simulink model "FullEKF_2010a"  (Simulink 6.6)
settings: Solver=FixedStepDiscrete  StartTime=0.0  StopTime=300  FixedStep=0.01  RelTol=1e-3
values from neighbouring files (symbols this model uses):
  initP = diag([1e-3 1e-3 1e-3 1e-6 1e-6 1e-6 1 1 1 5e-6 5e-6 5e-6 1e-8 1e-8 1e-8])    [FullEKF_init.m.m]
undefined symbols (not defined in the file or in its folder): DiscIntNeverNeededParam, gcbh, hwbcalib_subsystem
libraries: simulink x6, dspmtrx3 x4, dspinverses x1
(part 4 of 7)

== system FullEKF_2010a/Trajectory  Generator/Signals Conversions dtgen/Subsystem1 ==
  note: Equation for Transforming Geodetic Coordinate
      | to Rectangular (ECEF) coordinates:
      | (NIMA TR8350.2 Third Edition, 3 January 2000)
      |
      | Equation 4-14:
      | x_{ECEF} = (N + h)cos(\lambda)cos(\Lambda)
      | y_{ECEF} = (N + h)cos(\lambda)sin(\Lambda)
      | z_{ECEF} = ((b/a)^2N + h)sin(\lambda)
      |
      | Equation 4-15:
      | N = a / (1-e^2sin^2(\lambda))^{1/2}
      |
      | Where:
      | (\lambda, \Lambda, h) = geodetic coordinates (in meters & rad)
      | b/a = earth axis ratio
      | a = earth semi-major axis (in m)
      | e = earth first eccentricity
  geoToECEFLibInLon : Inport  OutDataType=fixdt(1,16,0)  OutScaling=[]
  geoToECEFLibInLat : Inport  Port=2  OutDataType=fixdt(1,16,0)  OutScaling=[]
  geoToECEFLibInAlt : Inport  Port=3  OutDataType=fixdt(1,16,0)  OutScaling=[]
  Math Function : Math  Operator=reciprocal  OutDataType=fixdt(1,16,0)  OutScaling=[]  SaturateOnIntegerOverflow=on
  Sqrt : Math  Operator=sqrt  OutDataType=fixdt(1,16,0)  OutScaling=[]  SaturateOnIntegerOverflow=on
  Trigonometric Function : Trigonometry  Operator=cos
  Trigonometric Function1 : Trigonometry  Operator=cos
  Trigonometric Function2 : Trigonometry
  Trigonometric Function3 : Trigonometry
  axisRatio : Gain  Tag=MBDLibrary v2007b.1  Gain=.996647189335^2  ParameterDataType=fixdt(1,16,0)  ParameterScaling=[]  OutDataType=fixdt(1,16,0)  OutScaling=[]  RndMeth=Zero  mask(Gain (MBDLibrary)){gain_mbdlib=.996647189335^2}
      mask prompts: gain_mbdlib "Gain"
      mask help: Multiplies the input by the gain.
      settings: OpenFcn=|
      | if exist('mbdlib_dialog')
      |    mbdlib_dialog(gcb,'open')
      | else
      |    open_system(gcb, 'mask')
      | end
      mask Help: The GAIN block multiplies the input by the gain value.  This block may accept any data types other than boolean.  The user must take care to not use a non-integer gain for int32/uint32 inputs.
      mask Display: disp([get_param(gcb, 'Gain') 'x'])
  bias : Bias  Tag=MBDLibrary v2007b.1  Bias=1  mask(Bias (MBDLibrary)){Bias_mbdlib=1}
      mask prompts: Bias_mbdlib "Bias"
      mask help: Add bias to input.
      settings: OpenFcn=|
      | if exist('mbdlib_dialog')
      |    mbdlib_dialog(gcb,'open')
      | else
      |    open_system(gcb, 'mask')
      | end
      settings: CloseFcn=|
      | if exist('mbdlib_bias')
      |    mbdlib_bias(gcb)
      | end
      mask Help: The BIAS block outputs the summation of an input with a specified constant.
      mask Display: disp(['x+1'])
  eqPlane : Product  Tag=MBDLibrary v2007b.1  OutDataType=fixdt(1,16,0)  OutScaling=[]  RndMeth=Zero  InputSameDT=on  mask(Product (MBDLibrary)){Inputs_mbdlib=2}
      mask prompts: Inputs_mbdlib "Number of Inputs"
      mask help: Multiplies inputs.
      settings: OpenFcn=|
      | if exist('mbdlib_dialog')
      |    mbdlib_dialog(gcb,'open')
      | else
      |    open_system(gcb, 'mask')
      | end
      mask Help: The PRODUCT block is used to multiply inputs.
  firstEccentricitySquared : Gain  Tag=MBDLibrary v2007b.1  Gain=-6.69437999014e-3  ParameterDataType=fixdt(1,16,0)  ParameterScaling=[]  OutDataType=fixdt(1,16,0)  OutScaling=[]  RndMeth=Zero  mask(Gain (MBDLibrary)){gain_mbdlib=-6.69437999014e-3}
      mask prompts: gain_mbdlib "Gain"
      mask help: Multiplies the input by the gain.
      settings: OpenFcn=|
      | if exist('mbdlib_dialog')
      |    mbdlib_dialog(gcb,'open')
      | else
      |    open_system(gcb, 'mask')
      | end
      mask Help: The GAIN block multiplies the input by the gain value.  This block may accept any data types other than boolean.  The user must take care to not use a non-integer gain for int32/uint32 inputs.
      mask Display: disp([get_param(gcb, 'Gain') 'x'])
  gain : Gain  Tag=MBDLibrary v2007b.1  Gain=6378137.0  ParameterDataType=fixdt(1,16,0)  ParameterScaling=[]  OutDataType=fixdt(1,16,0)  OutScaling=[]  RndMeth=Zero  mask(Gain (MBDLibrary)){gain_mbdlib=6378137.0}
      mask prompts: gain_mbdlib "Gain"
      mask help: Multiplies the input by the gain.
      settings: OpenFcn=|
      | if exist('mbdlib_dialog')
      |    mbdlib_dialog(gcb,'open')
      | else
      |    open_system(gcb, 'mask')
      | end
      mask Help: The GAIN block multiplies the input by the gain value.  This block may accept any data types other than boolean.  The user must take care to not use a non-integer gain for int32/uint32 inputs.
      mask Display: disp([get_param(gcb, 'Gain') 'x'])
  radius : Sum  Tag=MBDLibrary v2007b.1  OutDataType=fixdt(1,16,0)  OutScaling=[]  RndMeth=Zero  InputSameDT=on  mask(Sum (MBDLibrary)){inputs_mbdlib=++}
      mask prompts: inputs_mbdlib "List of signs"
      mask help: Adds values together.
      settings: OpenFcn=|
      | if exist('mbdlib_dialog')
      |    mbdlib_dialog(gcb,'open')
      | else
      |    open_system(gcb, 'mask')
      | end
      mask Help:
      | The SUM block is used to add or subtract  inputs.
      | The inputs may be specified as:
      |   (a) + or - for each port (i.e. ++-+)
      |   (b) An integer to indicate the number of ports to add
      | Note that the number of ports input to this block must be between 1 and 25.
      | When only 1 inport is selected, the block computes the summation of vector input elements and outputs a scalar.
  radius1 : Sum  Tag=MBDLibrary v2007b.1  OutDataType=fixdt(1,16,0)  OutScaling=[]  RndMeth=Zero  InputSameDT=on  mask(Sum (MBDLibrary)){inputs_mbdlib=++}
      mask prompts: inputs_mbdlib "List of signs"
      mask help: Adds values together.
      settings: OpenFcn=|
      | if exist('mbdlib_dialog')
      |    mbdlib_dialog(gcb,'open')
      | else
      |    open_system(gcb, 'mask')
      | end
      mask Help:
      | The SUM block is used to add or subtract  inputs.
      | The inputs may be specified as:
      |   (a) + or - for each port (i.e. ++-+)
      |   (b) An integer to indicate the number of ports to add
      | Note that the number of ports input to this block must be between 1 and 25.
      | When only 1 inport is selected, the block computes the summation of vector input elements and outputs a scalar.
  square : Subsystem  Tag=MBDLibrary v2007b.1
      settings: OpenFcn=|
      | if exist('mbdlib_dialog')
      |    mbdlib_dialog(gcb,'open')
      | else
      |    open_system(gcb, 'mask')
      | end
      mask Type: Square (MBDLibrary)
      mask Description: Squares the input.
      mask Help: The SQAURE block outputs the square of the input value.
      mask Display: disp('x^2', 'texmode', 'on')
  xECEF : Product  Tag=MBDLibrary v2007b.1  OutDataType=fixdt(1,16,0)  OutScaling=[]  RndMeth=Zero  InputSameDT=on  mask(Product (MBDLibrary)){Inputs_mbdlib=2}
      mask prompts: Inputs_mbdlib "Number of Inputs"
      mask help: Multiplies inputs.
      settings: OpenFcn=|
      | if exist('mbdlib_dialog')
      |    mbdlib_dialog(gcb,'open')
      | else
      |    open_system(gcb, 'mask')
      | end
      mask Help: The PRODUCT block is used to multiply inputs.
  yECEF : Product  Tag=MBDLibrary v2007b.1  OutDataType=fixdt(1,16,0)  OutScaling=[]  RndMeth=Zero  InputSameDT=on  mask(Product (MBDLibrary)){Inputs_mbdlib=2}
      mask prompts: Inputs_mbdlib "Number of Inputs"
      mask help: Multiplies inputs.
      settings: OpenFcn=|
      | if exist('mbdlib_dialog')
      |    mbdlib_dialog(gcb,'open')
      | else
      |    open_system(gcb, 'mask')
      | end
      mask Help: The PRODUCT block is used to multiply inputs.
  zECEF : Product  Tag=MBDLibrary v2007b.1  OutDataType=fixdt(1,16,0)  OutScaling=[]  RndMeth=Zero  InputSameDT=on  mask(Product (MBDLibrary)){Inputs_mbdlib=2}
      mask prompts: Inputs_mbdlib "Number of Inputs"
      mask help: Multiplies inputs.
      settings: OpenFcn=|
      | if exist('mbdlib_dialog')
      |    mbdlib_dialog(gcb,'open')
      | else
      |    open_system(gcb, 'mask')
      | end
      mask Help: The PRODUCT block is used to multiply inputs.
  geoToECEFLibOutX : Outport  OutDataType=fixdt(1,16,0)  OutScaling=[]
  geoToECEFLibOutY : Outport  Port=2  OutDataType=fixdt(1,16,0)  OutScaling=[]
  geoToECEFLibOutZ : Outport  Port=3  OutDataType=fixdt(1,16,0)  OutScaling=[]
  wires:
  Trigonometric Function3/1 -> zECEF/2, square/1(squareLibIn)
  zECEF/1 -> geoToECEFLibOutZ/1
  yECEF/1 -> geoToECEFLibOutY/1
  xECEF/1 -> geoToECEFLibOutX/1
  radius1/1 -> zECEF/1
  eqPlane/1 -> yECEF/2, xECEF/1
  Trigonometric Function2/1 -> yECEF/1
  geoToECEFLibInLon/1 -> Trigonometric Function1/1, Trigonometric Function2/1
  axisRatio/1 -> radius1/2
  geoToECEFLibInAlt/1 -> radius1/1, radius/2
  gain/1 -> axisRatio/1, radius/1
  Trigonometric Function/1 -> eqPlane/1
  Trigonometric Function1/1 -> xECEF/2
  radius/1 -> eqPlane/2
  bias/1 -> Sqrt/1
  firstEccentricitySquared/1 -> bias/1
  square/1(squareLibOut) -> firstEccentricitySquared/1
  geoToECEFLibInLat/1 -> Trigonometric Function/1, Trigonometric Function3/1
  Sqrt/1 -> Math Function/1
  Math Function/1 -> gain/1

== system FullEKF_2010a/EKF/MeasureVector/GPS/Subsystem1 ==
  note: Equation for Transforming Geodetic Coordinate
      | to Rectangular (ECEF) coordinates:
      | (NIMA TR8350.2 Third Edition, 3 January 2000)
      |
      | Equation 4-14:
      | x_{ECEF} = (N + h)cos(\lambda)cos(\Lambda)
      | y_{ECEF} = (N + h)cos(\lambda)sin(\Lambda)
      | z_{ECEF} = ((b/a)^2N + h)sin(\lambda)
      |
      | Equation 4-15:
      | N = a / (1-e^2sin^2(\lambda))^{1/2}
      |
      | Where:
      | (\lambda, \Lambda, h) = geodetic coordinates (in meters & rad)
      | b/a = earth axis ratio
      | a = earth semi-major axis (in m)
      | e = earth first eccentricity
  geoToECEFLibInLon : Inport  OutDataType=fixdt(1,16,0)  OutScaling=[]
  geoToECEFLibInLat : Inport  Port=2  OutDataType=fixdt(1,16,0)  OutScaling=[]
  geoToECEFLibInAlt : Inport  Port=3  OutDataType=fixdt(1,16,0)  OutScaling=[]
  Math Function : Math  Operator=reciprocal  OutDataType=fixdt(1,16,0)  OutScaling=[]  SaturateOnIntegerOverflow=on
  Sqrt : Math  Operator=sqrt  OutDataType=fixdt(1,16,0)  OutScaling=[]  SaturateOnIntegerOverflow=on
  Trigonometric Function : Trigonometry  Operator=cos
  Trigonometric Function1 : Trigonometry  Operator=cos
  Trigonometric Function2 : Trigonometry
  Trigonometric Function3 : Trigonometry
  axisRatio : Gain  Tag=MBDLibrary v2007b.1  Gain=.996647189335^2  ParameterDataType=fixdt(1,16,0)  ParameterScaling=[]  OutDataType=fixdt(1,16,0)  OutScaling=[]  RndMeth=Zero  mask(Gain (MBDLibrary)){gain_mbdlib=.996647189335^2}
      mask prompts: gain_mbdlib "Gain"
      mask help: Multiplies the input by the gain.
      settings: OpenFcn=|
      | if exist('mbdlib_dialog')
      |    mbdlib_dialog(gcb,'open')
      | else
      |    open_system(gcb, 'mask')
      | end
      mask Help: The GAIN block multiplies the input by the gain value.  This block may accept any data types other than boolean.  The user must take care to not use a non-integer gain for int32/uint32 inputs.
      mask Display: disp([get_param(gcb, 'Gain') 'x'])
  bias : Bias  Tag=MBDLibrary v2007b.1  Bias=1  mask(Bias (MBDLibrary)){Bias_mbdlib=1}
      mask prompts: Bias_mbdlib "Bias"
      mask help: Add bias to input.
      settings: OpenFcn=|
      | if exist('mbdlib_dialog')
      |    mbdlib_dialog(gcb,'open')
      | else
      |    open_system(gcb, 'mask')
      | end
      settings: CloseFcn=|
      | if exist('mbdlib_bias')
      |    mbdlib_bias(gcb)
      | end
      mask Help: The BIAS block outputs the summation of an input with a specified constant.
      mask Display: disp(['x+1'])
  eqPlane : Product  Tag=MBDLibrary v2007b.1  OutDataType=fixdt(1,16,0)  OutScaling=[]  RndMeth=Zero  InputSameDT=on  mask(Product (MBDLibrary)){Inputs_mbdlib=2}
      mask prompts: Inputs_mbdlib "Number of Inputs"
      mask help: Multiplies inputs.
      settings: OpenFcn=|
      | if exist('mbdlib_dialog')
      |    mbdlib_dialog(gcb,'open')
      | else
      |    open_system(gcb, 'mask')
      | end
      mask Help: The PRODUCT block is used to multiply inputs.
  firstEccentricitySquared : Gain  Tag=MBDLibrary v2007b.1  Gain=-6.69437999014e-3  ParameterDataType=fixdt(1,16,0)  ParameterScaling=[]  OutDataType=fixdt(1,16,0)  OutScaling=[]  RndMeth=Zero  mask(Gain (MBDLibrary)){gain_mbdlib=-6.69437999014e-3}
      mask prompts: gain_mbdlib "Gain"
      mask help: Multiplies the input by the gain.
      settings: OpenFcn=|
      | if exist('mbdlib_dialog')
      |    mbdlib_dialog(gcb,'open')
      | else
      |    open_system(gcb, 'mask')
      | end
      mask Help: The GAIN block multiplies the input by the gain value.  This block may accept any data types other than boolean.  The user must take care to not use a non-integer gain for int32/uint32 inputs.
      mask Display: disp([get_param(gcb, 'Gain') 'x'])
  gain : Gain  Tag=MBDLibrary v2007b.1  Gain=6378137.0  ParameterDataType=fixdt(1,16,0)  ParameterScaling=[]  OutDataType=fixdt(1,16,0)  OutScaling=[]  RndMeth=Zero  mask(Gain (MBDLibrary)){gain_mbdlib=6378137.0}
      mask prompts: gain_mbdlib "Gain"
      mask help: Multiplies the input by the gain.
      settings: OpenFcn=|
      | if exist('mbdlib_dialog')
      |    mbdlib_dialog(gcb,'open')
      | else
      |    open_system(gcb, 'mask')
      | end
      mask Help: The GAIN block multiplies the input by the gain value.  This block may accept any data types other than boolean.  The user must take care to not use a non-integer gain for int32/uint32 inputs.
      mask Display: disp([get_param(gcb, 'Gain') 'x'])
  radius : Sum  Tag=MBDLibrary v2007b.1  OutDataType=fixdt(1,16,0)  OutScaling=[]  RndMeth=Zero  InputSameDT=on  mask(Sum (MBDLibrary)){inputs_mbdlib=++}
      mask prompts: inputs_mbdlib "List of signs"
      mask help: Adds values together.
      settings: OpenFcn=|
      | if exist('mbdlib_dialog')
      |    mbdlib_dialog(gcb,'open')
      | else
      |    open_system(gcb, 'mask')
      | end
      mask Help:
      | The SUM block is used to add or subtract  inputs.
      | The inputs may be specified as:
      |   (a) + or - for each port (i.e. ++-+)
      |   (b) An integer to indicate the number of ports to add
      | Note that the number of ports input to this block must be between 1 and 25.
      | When only 1 inport is selected, the block computes the summation of vector input elements and outputs a scalar.
  radius1 : Sum  Tag=MBDLibrary v2007b.1  OutDataType=fixdt(1,16,0)  OutScaling=[]  RndMeth=Zero  InputSameDT=on  mask(Sum (MBDLibrary)){inputs_mbdlib=++}
      mask prompts: inputs_mbdlib "List of signs"
      mask help: Adds values together.
      settings: OpenFcn=|
      | if exist('mbdlib_dialog')
      |    mbdlib_dialog(gcb,'open')
      | else
      |    open_system(gcb, 'mask')
      | end
      mask Help:
      | The SUM block is used to add or subtract  inputs.
      | The inputs may be specified as:
      |   (a) + or - for each port (i.e. ++-+)
      |   (b) An integer to indicate the number of ports to add
      | Note that the number of ports input to this block must be between 1 and 25.
      | When only 1 inport is selected, the block computes the summation of vector input elements and outputs a scalar.
  square : Subsystem  Tag=MBDLibrary v2007b.1
      settings: OpenFcn=|
      | if exist('mbdlib_dialog')
      |    mbdlib_dialog(gcb,'open')
      | else
      |    open_system(gcb, 'mask')
      | end
      mask Type: Square (MBDLibrary)
      mask Description: Squares the input.
      mask Help: The SQAURE block outputs the square of the input value.
      mask Display: disp('x^2', 'texmode', 'on')
  xECEF : Product  Tag=MBDLibrary v2007b.1  OutDataType=fixdt(1,16,0)  OutScaling=[]  RndMeth=Zero  InputSameDT=on  mask(Product (MBDLibrary)){Inputs_mbdlib=2}
      mask prompts: Inputs_mbdlib "Number of Inputs"
      mask help: Multiplies inputs.
      settings: OpenFcn=|
      | if exist('mbdlib_dialog')
      |    mbdlib_dialog(gcb,'open')
      | else
      |    open_system(gcb, 'mask')
      | end
      mask Help: The PRODUCT block is used to multiply inputs.
  yECEF : Product  Tag=MBDLibrary v2007b.1  OutDataType=fixdt(1,16,0)  OutScaling=[]  RndMeth=Zero  InputSameDT=on  mask(Product (MBDLibrary)){Inputs_mbdlib=2}
      mask prompts: Inputs_mbdlib "Number of Inputs"
      mask help: Multiplies inputs.
      settings: OpenFcn=|
      | if exist('mbdlib_dialog')
      |    mbdlib_dialog(gcb,'open')
      | else
      |    open_system(gcb, 'mask')
      | end
      mask Help: The PRODUCT block is used to multiply inputs.
  zECEF : Product  Tag=MBDLibrary v2007b.1  OutDataType=fixdt(1,16,0)  OutScaling=[]  RndMeth=Zero  InputSameDT=on  mask(Product (MBDLibrary)){Inputs_mbdlib=2}
      mask prompts: Inputs_mbdlib "Number of Inputs"
      mask help: Multiplies inputs.
      settings: OpenFcn=|
      | if exist('mbdlib_dialog')
      |    mbdlib_dialog(gcb,'open')
      | else
      |    open_system(gcb, 'mask')
      | end
      mask Help: The PRODUCT block is used to multiply inputs.
  geoToECEFLibOutX : Outport  OutDataType=fixdt(1,16,0)  OutScaling=[]
  geoToECEFLibOutY : Outport  Port=2  OutDataType=fixdt(1,16,0)  OutScaling=[]
  geoToECEFLibOutZ : Outport  Port=3  OutDataType=fixdt(1,16,0)  OutScaling=[]
  wires:
  Trigonometric Function3/1 -> zECEF/2, square/1(squareLibIn)
  zECEF/1 -> geoToECEFLibOutZ/1
  yECEF/1 -> geoToECEFLibOutY/1
  xECEF/1 -> geoToECEFLibOutX/1
  radius1/1 -> zECEF/1
  eqPlane/1 -> yECEF/2, xECEF/1
  Trigonometric Function2/1 -> yECEF/1
  geoToECEFLibInLon/1 -> Trigonometric Function1/1, Trigonometric Function2/1
  axisRatio/1 -> radius1/2
  geoToECEFLibInAlt/1 -> radius1/1, radius/2
  gain/1 -> axisRatio/1, radius/1
  Trigonometric Function/1 -> eqPlane/1
  Trigonometric Function1/1 -> xECEF/2
  radius/1 -> eqPlane/2
  bias/1 -> Sqrt/1
  firstEccentricitySquared/1 -> bias/1
  square/1(squareLibOut) -> firstEccentricitySquared/1
  geoToECEFLibInLat/1 -> Trigonometric Function/1, Trigonometric Function3/1
  Sqrt/1 -> Math Function/1
  Math Function/1 -> gain/1

== system FullEKF_2010a/EKF/MeasureVector/GPS/Subsystem2 ==
  note: Equation for Transforming Geodetic Coordinate
      | to Rectangular (ECEF) coordinates:
      | (NIMA TR8350.2 Third Edition, 3 January 2000)
      |
      | Equation 4-14:
      | x_{ECEF} = (N + h)cos(\lambda)cos(\Lambda)
      | y_{ECEF} = (N + h)cos(\lambda)sin(\Lambda)
      | z_{ECEF} = ((b/a)^2N + h)sin(\lambda)
      |
      | Equation 4-15:
      | N = a / (1-e^2sin^2(\lambda))^{1/2}
      |
      | Where:
      | (\lambda, \Lambda, h) = geodetic coordinates (in meters & rad)
      | b/a = earth axis ratio
      | a = earth semi-major axis (in m)
      | e = earth first eccentricity
  geoToECEFLibInLon : Inport  OutDataType=fixdt(1,16,0)  OutScaling=[]
  geoToECEFLibInLat : Inport  Port=2  OutDataType=fixdt(1,16,0)  OutScaling=[]
  geoToECEFLibInAlt : Inport  Port=3  OutDataType=fixdt(1,16,0)  OutScaling=[]
  Math Function : Math  Operator=reciprocal  OutDataType=fixdt(1,16,0)  OutScaling=[]  SaturateOnIntegerOverflow=on
  Sqrt : Math  Operator=sqrt  OutDataType=fixdt(1,16,0)  OutScaling=[]  SaturateOnIntegerOverflow=on
  Trigonometric Function : Trigonometry  Operator=cos
  Trigonometric Function1 : Trigonometry  Operator=cos
  Trigonometric Function2 : Trigonometry
  Trigonometric Function3 : Trigonometry
  axisRatio : Gain  Tag=MBDLibrary v2007b.1  Gain=.996647189335^2  ParameterDataType=fixdt(1,16,0)  ParameterScaling=[]  OutDataType=fixdt(1,16,0)  OutScaling=[]  RndMeth=Zero  mask(Gain (MBDLibrary)){gain_mbdlib=.996647189335^2}
      mask prompts: gain_mbdlib "Gain"
      mask help: Multiplies the input by the gain.
      settings: OpenFcn=|
      | if exist('mbdlib_dialog')
      |    mbdlib_dialog(gcb,'open')
      | else
      |    open_system(gcb, 'mask')
      | end
      mask Help: The GAIN block multiplies the input by the gain value.  This block may accept any data types other than boolean.  The user must take care to not use a non-integer gain for int32/uint32 inputs.
      mask Display: disp([get_param(gcb, 'Gain') 'x'])
  bias : Bias  Tag=MBDLibrary v2007b.1  Bias=1  mask(Bias (MBDLibrary)){Bias_mbdlib=1}
      mask prompts: Bias_mbdlib "Bias"
      mask help: Add bias to input.
      settings: OpenFcn=|
      | if exist('mbdlib_dialog')
      |    mbdlib_dialog(gcb,'open')
      | else
      |    open_system(gcb, 'mask')
      | end
      settings: CloseFcn=|
      | if exist('mbdlib_bias')
      |    mbdlib_bias(gcb)
      | end
      mask Help: The BIAS block outputs the summation of an input with a specified constant.
      mask Display: disp(['x+1'])
  eqPlane : Product  Tag=MBDLibrary v2007b.1  OutDataType=fixdt(1,16,0)  OutScaling=[]  RndMeth=Zero  InputSameDT=on  mask(Product (MBDLibrary)){Inputs_mbdlib=2}
      mask prompts: Inputs_mbdlib "Number of Inputs"
      mask help: Multiplies inputs.
      settings: OpenFcn=|
      | if exist('mbdlib_dialog')
      |    mbdlib_dialog(gcb,'open')
      | else
      |    open_system(gcb, 'mask')
      | end
      mask Help: The PRODUCT block is used to multiply inputs.
  firstEccentricitySquared : Gain  Tag=MBDLibrary v2007b.1  Gain=-6.69437999014e-3  ParameterDataType=fixdt(1,16,0)  ParameterScaling=[]  OutDataType=fixdt(1,16,0)  OutScaling=[]  RndMeth=Zero  mask(Gain (MBDLibrary)){gain_mbdlib=-6.69437999014e-3}
      mask prompts: gain_mbdlib "Gain"
      mask help: Multiplies the input by the gain.
      settings: OpenFcn=|
      | if exist('mbdlib_dialog')
      |    mbdlib_dialog(gcb,'open')
      | else
      |    open_system(gcb, 'mask')
      | end
      mask Help: The GAIN block multiplies the input by the gain value.  This block may accept any data types other than boolean.  The user must take care to not use a non-integer gain for int32/uint32 inputs.
      mask Display: disp([get_param(gcb, 'Gain') 'x'])
  gain : Gain  Tag=MBDLibrary v2007b.1  Gain=6378137.0  ParameterDataType=fixdt(1,16,0)  ParameterScaling=[]  OutDataType=fixdt(1,16,0)  OutScaling=[]  RndMeth=Zero  mask(Gain (MBDLibrary)){gain_mbdlib=6378137.0}
      mask prompts: gain_mbdlib "Gain"
      mask help: Multiplies the input by the gain.
      settings: OpenFcn=|
      | if exist('mbdlib_dialog')
      |    mbdlib_dialog(gcb,'open')
      | else
      |    open_system(gcb, 'mask')
      | end
      mask Help: The GAIN block multiplies the input by the gain value.  This block may accept any data types other than boolean.  The user must take care to not use a non-integer gain for int32/uint32 inputs.
      mask Display: disp([get_param(gcb, 'Gain') 'x'])
  radius : Sum  Tag=MBDLibrary v2007b.1  OutDataType=fixdt(1,16,0)  OutScaling=[]  RndMeth=Zero  InputSameDT=on  mask(Sum (MBDLibrary)){inputs_mbdlib=++}
      mask prompts: inputs_mbdlib "List of signs"
      mask help: Adds values together.
      settings: OpenFcn=|
      | if exist('mbdlib_dialog')
      |    mbdlib_dialog(gcb,'open')
      | else
      |    open_system(gcb, 'mask')
      | end
      mask Help:
      | The SUM block is used to add or subtract  inputs.
      | The inputs may be specified as:
      |   (a) + or - for each port (i.e. ++-+)
      |   (b) An integer to indicate the number of ports to add
      | Note that the number of ports input to this block must be between 1 and 25.
      | When only 1 inport is selected, the block computes the summation of vector input elements and outputs a scalar.
  radius1 : Sum  Tag=MBDLibrary v2007b.1  OutDataType=fixdt(1,16,0)  OutScaling=[]  RndMeth=Zero  InputSameDT=on  mask(Sum (MBDLibrary)){inputs_mbdlib=++}
      mask prompts: inputs_mbdlib "List of signs"
      mask help: Adds values together.
      settings: OpenFcn=|
      | if exist('mbdlib_dialog')
      |    mbdlib_dialog(gcb,'open')
      | else
      |    open_system(gcb, 'mask')
      | end
      mask Help:
      | The SUM block is used to add or subtract  inputs.
      | The inputs may be specified as:
      |   (a) + or - for each port (i.e. ++-+)
      |   (b) An integer to indicate the number of ports to add
      | Note that the number of ports input to this block must be between 1 and 25.
      | When only 1 inport is selected, the block computes the summation of vector input elements and outputs a scalar.
  square : Subsystem  Tag=MBDLibrary v2007b.1
      settings: OpenFcn=|
      | if exist('mbdlib_dialog')
      |    mbdlib_dialog(gcb,'open')
      | else
      |    open_system(gcb, 'mask')
      | end
      mask Type: Square (MBDLibrary)
      mask Description: Squares the input.
      mask Help: The SQAURE block outputs the square of the input value.
      mask Display: disp('x^2', 'texmode', 'on')
  xECEF : Product  Tag=MBDLibrary v2007b.1  OutDataType=fixdt(1,16,0)  OutScaling=[]  RndMeth=Zero  InputSameDT=on  mask(Product (MBDLibrary)){Inputs_mbdlib=2}
      mask prompts: Inputs_mbdlib "Number of Inputs"
      mask help: Multiplies inputs.
      settings: OpenFcn=|
      | if exist('mbdlib_dialog')
      |    mbdlib_dialog(gcb,'open')
      | else
      |    open_system(gcb, 'mask')
      | end
      mask Help: The PRODUCT block is used to multiply inputs.
  yECEF : Product  Tag=MBDLibrary v2007b.1  OutDataType=fixdt(1,16,0)  OutScaling=[]  RndMeth=Zero  InputSameDT=on  mask(Product (MBDLibrary)){Inputs_mbdlib=2}
      mask prompts: Inputs_mbdlib "Number of Inputs"
      mask help: Multiplies inputs.
      settings: OpenFcn=|
      | if exist('mbdlib_dialog')
      |    mbdlib_dialog(gcb,'open')
      | else
      |    open_system(gcb, 'mask')
      | end
      mask Help: The PRODUCT block is used to multiply inputs.
  zECEF : Product  Tag=MBDLibrary v2007b.1  OutDataType=fixdt(1,16,0)  OutScaling=[]  RndMeth=Zero  InputSameDT=on  mask(Product (MBDLibrary)){Inputs_mbdlib=2}
      mask prompts: Inputs_mbdlib "Number of Inputs"
      mask help: Multiplies inputs.
      settings: OpenFcn=|
      | if exist('mbdlib_dialog')
      |    mbdlib_dialog(gcb,'open')
      | else
      |    open_system(gcb, 'mask')
      | end
      mask Help: The PRODUCT block is used to multiply inputs.
  geoToECEFLibOutX : Outport  OutDataType=fixdt(1,16,0)  OutScaling=[]
  geoToECEFLibOutY : Outport  Port=2  OutDataType=fixdt(1,16,0)  OutScaling=[]
  geoToECEFLibOutZ : Outport  Port=3  OutDataType=fixdt(1,16,0)  OutScaling=[]
  wires:
  Trigonometric Function3/1 -> zECEF/2, square/1(squareLibIn)
  zECEF/1 -> geoToECEFLibOutZ/1
  yECEF/1 -> geoToECEFLibOutY/1
  xECEF/1 -> geoToECEFLibOutX/1
  radius1/1 -> zECEF/1
  eqPlane/1 -> yECEF/2, xECEF/1
  Trigonometric Function2/1 -> yECEF/1
  geoToECEFLibInLon/1 -> Trigonometric Function1/1, Trigonometric Function2/1
  axisRatio/1 -> radius1/2
  geoToECEFLibInAlt/1 -> radius1/1, radius/2
  gain/1 -> axisRatio/1, radius/1
  Trigonometric Function/1 -> eqPlane/1
  Trigonometric Function1/1 -> xECEF/2
  radius/1 -> eqPlane/2
  bias/1 -> Sqrt/1
  firstEccentricitySquared/1 -> bias/1
  square/1(squareLibOut) -> firstEccentricitySquared/1
  geoToECEFLibInLat/1 -> Trigonometric Function/1, Trigonometric Function3/1
  Sqrt/1 -> Math Function/1
  Math Function/1 -> gain/1

== system FullEKF_2010a/INS/Attitude update/Stage2/Subsystem ==
  Quat : Inport  PortDimensions=4  OutDataType=fixdt(1,16,0)  OutScaling=[]
  Subsystem : Subsystem
  a11 : Subsystem  InitFcn=%hwbcalib_subsystem(gcbh,99);
      settings: AttributesFormatString=(Page 13)  CopyFcn=hwbcalib_copyfcn(gcbh);  DeleteFcn=hwbcalib_subsystem(gcbh,'delete');
      mask Type: Subsystem (HW)
      mask Display:
      | port_label('input',1,'quat');
      | port_label('output',1,'a11');
  a12 : Subsystem  InitFcn=%hwbcalib_subsystem(gcbh,99);
      settings: AttributesFormatString=(Page 14)  CopyFcn=hwbcalib_copyfcn(gcbh);  DeleteFcn=hwbcalib_subsystem(gcbh,'delete');
      mask Type: Subsystem (HW)
      mask Display:
      | port_label('input',1,'quat');
      | port_label('output',1,'a12');
  a13 : Subsystem  InitFcn=%hwbcalib_subsystem(gcbh,99);
      settings: AttributesFormatString=(Page 15)  CopyFcn=hwbcalib_copyfcn(gcbh);  DeleteFcn=hwbcalib_subsystem(gcbh,'delete');
      mask Type: Subsystem (HW)
      mask Display:
      | port_label('input',1,'quat');
      | port_label('output',1,'a13');
  a21 : Subsystem  InitFcn=%hwbcalib_subsystem(gcbh,99);
      settings: AttributesFormatString=(Page 16)  CopyFcn=hwbcalib_copyfcn(gcbh);  DeleteFcn=hwbcalib_subsystem(gcbh,'delete');
      mask Type: Subsystem (HW)
      mask Display:
      | port_label('input',1,'quat');
      | port_label('output',1,'a21');
  a22 : Subsystem  InitFcn=%hwbcalib_subsystem(gcbh,99);
      settings: AttributesFormatString=(Page 17)  CopyFcn=hwbcalib_copyfcn(gcbh);  DeleteFcn=hwbcalib_subsystem(gcbh,'delete');
      mask Type: Subsystem (HW)
      mask Display:
      | port_label('input',1,'quat');
      | port_label('output',1,'a22');
  a23 : Subsystem  InitFcn=%hwbcalib_subsystem(gcbh,99);
      settings: AttributesFormatString=(Page 18)  CopyFcn=hwbcalib_copyfcn(gcbh);  DeleteFcn=hwbcalib_subsystem(gcbh,'delete');
      mask Type: Subsystem (HW)
      mask Display:
      | port_label('input',1,'quat');
      | port_label('output',1,'a23');
  a31 : Subsystem  InitFcn=%hwbcalib_subsystem(gcbh,99);
      settings: AttributesFormatString=(Page 19)  CopyFcn=hwbcalib_copyfcn(gcbh);  DeleteFcn=hwbcalib_subsystem(gcbh,'delete');
      mask Type: Subsystem (HW)
      mask Display:
      | port_label('input',1,'quat');
      | port_label('output',1,'a31');
  a32 : Subsystem  InitFcn=%hwbcalib_subsystem(gcbh,99);
      settings: AttributesFormatString=(Page 20)  CopyFcn=hwbcalib_copyfcn(gcbh);  DeleteFcn=hwbcalib_subsystem(gcbh,'delete');
      mask Type: Subsystem (HW)
      mask Display:
      | port_label('input',1,'quat');
      | port_label('output',1,'a32');
  a33 : Subsystem  InitFcn=%hwbcalib_subsystem(gcbh,99);
      settings: AttributesFormatString=(Page 21)  CopyFcn=hwbcalib_copyfcn(gcbh);  DeleteFcn=hwbcalib_subsystem(gcbh,'delete');
      mask Type: Subsystem (HW)
      mask Display:
      | port_label('input',1,'quat');
      | port_label('output',1,'a33');
  quat normalize : Subsystem
  DCM : Outport  PortDimensions=[3,3]  OutDataType=fixdt(1,16,0)  OutScaling=[]  InitialOutput=0
  wires:
  Quat/1 -> quat normalize/1(q)
  Subsystem/1(Matrix) -> DCM/1
  quat normalize/1(normal(q)) -> a11/1(quat), a21/1(quat), a31/1(quat), a12/1(quat), a22/1(quat), a32/1(quat), a13/1(quat), a23/1(quat), a33/1(quat)
  a11/1(a11) -> Subsystem/1(M11)
  a21/1(a21) -> Subsystem/2(M21)
  a31/1(a31) -> Subsystem/3(M31)
  a12/1(a12) -> Subsystem/4(M12)
  a22/1(a22) -> Subsystem/5(M22)
  a32/1(a32) -> Subsystem/6(M32)
  a13/1(a13) -> Subsystem/7(M13)
  a23/1(a23) -> Subsystem/8(M23)
  a33/1(a33) -> Subsystem/9(M33)

== system FullEKF_2010a/INS/Attitude update/Stage2/Subsystem1 ==
  note: Direction Cosine Matrix to Euler Angle Conversion
      |
      | Roll = ATAN2(SIN(PHI)*COS(THETA),COS(PHI)*COS(THETA))
      | Pitch = ASIN(SIN(THETA))
      | Yaw = ATAN2(SIN(PSI)*COS(THETA),COS(PSI)*COS(THETA))
  1 : Inport  PortDimensions=[3 3]  DataType=double  OutDataType=fixdt(1,16,0)  OutScaling=[]
  Reshape : Reshape  OutputDimensionality=Customize  OutputDimensions=[9,1]
  Trigonometric Function : Trigonometry  Operator=asin
  Trigonometric Function1 : Trigonometry  Operator=atan2
  Trigonometric Function2 : Trigonometry  Operator=atan2
  gain : Gain  Tag=MBDLibrary v2007b.1  Gain=-1  ParameterDataType=fixdt(1,16,0)  ParameterScaling=[]  OutDataType=fixdt(1,16,0)  OutScaling=[]  RndMeth=Zero  mask(Gain (MBDLibrary)){gain_mbdlib=-1}
      mask prompts: gain_mbdlib "Gain"
      mask help: Multiplies the input by the gain.
      settings: OpenFcn=|
      | if exist('mbdlib_dialog')
      |    mbdlib_dialog(gcb,'open')
      | else
      |    open_system(gcb, 'mask')
      | end
      mask Help: The GAIN block multiplies the input by the gain value.  This block may accept any data types other than boolean.  The user must take care to not use a non-integer gain for int32/uint32 inputs.
      mask Display: disp([get_param(gcb, 'Gain') 'x'])
  limit : Saturate  Tag=MBDLibrary v2007b.1  UpperLimit=1  LowerLimit=-1  ZeroCross=off  mask(Limit (MBDLibrary)){UpperLimit_mbdlib=1, LowerLimit_mbdlib=-1}
      mask prompts: UpperLimit_mbdlib "Upper Limit"; LowerLimit_mbdlib "Lower Limit"
      mask help: Provides upper and lower bounds for a signal.
      settings: AttributesFormatString={%<LowerLimit> to %<UpperLimit>}
      settings: OpenFcn=|
      | if exist('mbdlib_dialog')
      |    mbdlib_dialog(gcb,'open')
      | else
      |    open_system(gcb, 'mask')
      | end
      mask Help: The  LIMITER block provides upper and lower bounds for a signal.  If the input is between the boundaries, it is passed directly to the output.  If the input is greater than the upper bound, it will be output as the upper boundary value.  If the input is less than the lower bound, it will be output as the lower boundary value.  This block will accept any except Boolean inputs, and is vectorized.
  selector : Selector  Tag=MBDLibrary v2007b.1  IndexOptions=Index vector (dialog)  Indices=8  OutputSizes=1  InputPortWidth=9  mask(Mux Selector (MBDLibrary)){InputPortWidth_mbdlib=9, Indices_mbdlib=8}
      mask prompts: InputPortWidth_mbdlib "Input Port Width"; Indices_mbdlib "Output Indices"
      mask help: Changes the order of the inputs.
      settings: OpenFcn=|
      | if exist('mbdlib_dialog')
      |    mbdlib_dialog(gcb,'open')
      | else
      |    open_system(gcb, 'mask')
      | end
      settings: CloseFcn=|
      | if exist('mbdlib_selector')
      |    mbdlib_selector(gcb)
      | end
      mask Help: The SELECTOR block is a MULTIPLEXED SELECTOR block, used to change the input/output order of a multiplexed data stream.
      mask Display:
      | port_label('input', 1,'[9]')
      | text(1.0,0.5,'8', 'horizontalAlignment', 'right')
  selector1 : Selector  Tag=MBDLibrary v2007b.1  IndexOptions=Index vector (dialog)  Indices=9  OutputSizes=1  InputPortWidth=9  mask(Mux Selector (MBDLibrary)){InputPortWidth_mbdlib=9, Indices_mbdlib=9}
      mask prompts: InputPortWidth_mbdlib "Input Port Width"; Indices_mbdlib "Output Indices"
      mask help: Changes the order of the inputs.
      settings: OpenFcn=|
      | if exist('mbdlib_dialog')
      |    mbdlib_dialog(gcb,'open')
      | else
      |    open_system(gcb, 'mask')
      | end
      settings: CloseFcn=|
      | if exist('mbdlib_selector')
      |    mbdlib_selector(gcb)
      | end
      mask Help: The SELECTOR block is a MULTIPLEXED SELECTOR block, used to change the input/output order of a multiplexed data stream.
      mask Display:
      | port_label('input', 1,'[9]')
      | text(1.0,0.5,'9', 'horizontalAlignment', 'right')
  selector2 : Selector  Tag=MBDLibrary v2007b.1  IndexOptions=Index vector (dialog)  Indices=7  OutputSizes=1  InputPortWidth=9  mask(Mux Selector (MBDLibrary)){InputPortWidth_mbdlib=9, Indices_mbdlib=7}
      mask prompts: InputPortWidth_mbdlib "Input Port Width"; Indices_mbdlib "Output Indices"
      mask help: Changes the order of the inputs.
      settings: OpenFcn=|
      | if exist('mbdlib_dialog')
      |    mbdlib_dialog(gcb,'open')
      | else
      |    open_system(gcb, 'mask')
      | end
      settings: CloseFcn=|
      | if exist('mbdlib_selector')
      |    mbdlib_selector(gcb)
      | end
      mask Help: The SELECTOR block is a MULTIPLEXED SELECTOR block, used to change the input/output order of a multiplexed data stream.
      mask Display:
      | port_label('input', 1,'[9]')
      | text(1.0,0.5,'7', 'horizontalAlignment', 'right')
  selector3 : Selector  Tag=MBDLibrary v2007b.1  IndexOptions=Index vector (dialog)  Indices=4  OutputSizes=1  InputPortWidth=9  mask(Mux Selector (MBDLibrary)){InputPortWidth_mbdlib=9, Indices_mbdlib=4}
      mask prompts: InputPortWidth_mbdlib "Input Port Width"; Indices_mbdlib "Output Indices"
      mask help: Changes the order of the inputs.
      settings: OpenFcn=|
      | if exist('mbdlib_dialog')
      |    mbdlib_dialog(gcb,'open')
      | else
      |    open_system(gcb, 'mask')
      | end
      settings: CloseFcn=|
      | if exist('mbdlib_selector')
      |    mbdlib_selector(gcb)
      | end
      mask Help: The SELECTOR block is a MULTIPLEXED SELECTOR block, used to change the input/output order of a multiplexed data stream.
      mask Display:
      | port_label('input', 1,'[9]')
      | text(1.0,0.5,'4', 'horizontalAlignment', 'right')
  selector4 : Selector  Tag=MBDLibrary v2007b.1  IndexOptions=Index vector (dialog)  Indices=1  OutputSizes=1  InputPortWidth=9  mask(Mux Selector (MBDLibrary)){InputPortWidth_mbdlib=9, Indices_mbdlib=1}
      mask prompts: InputPortWidth_mbdlib "Input Port Width"; Indices_mbdlib "Output Indices"
      mask help: Changes the order of the inputs.
      settings: OpenFcn=|
      | if exist('mbdlib_dialog')
      |    mbdlib_dialog(gcb,'open')
      | else
      |    open_system(gcb, 'mask')
      | end
      settings: CloseFcn=|
      | if exist('mbdlib_selector')
      |    mbdlib_selector(gcb)
      | end
      mask Help: The SELECTOR block is a MULTIPLEXED SELECTOR block, used to change the input/output order of a multiplexed data stream.
      mask Display:
      | port_label('input', 1,'[9]')
      | text(1.0,0.5,'1', 'horizontalAlignment', 'right')
  2 : Outport  OutDataType=fixdt(1,16,0)  OutScaling=[]  InitialOutput=0
  3 : Outport  Port=2  OutDataType=fixdt(1,16,0)  OutScaling=[]  InitialOutput=0
  4 : Outport  Port=3  OutDataType=fixdt(1,16,0)  OutScaling=[]  InitialOutput=0
  wires:
  gain/1 -> selector2/1
  limit/1 -> Trigonometric Function/1
  1/1 -> Reshape/1
  Reshape/1 -> gain/1, selector1/1, selector/1, selector4/1, selector3/1
  selector2/1 -> limit/1
  selector/1 -> Trigonometric Function1/1
  selector1/1 -> Trigonometric Function1/2
  selector3/1 -> Trigonometric Function2/1
  selector4/1 -> Trigonometric Function2/2
  Trigonometric Function1/1 -> 2/1
  Trigonometric Function/1 -> 3/1
  Trigonometric Function2/1 -> 4/1
